simulink model "untitled"  (R2022b)
settings: Solver=ode15s  StartTime=0.0  StopTime=10  RelTol=1e-3
settings Model: Creator=Cmos  LastModifiedBy=Cmos

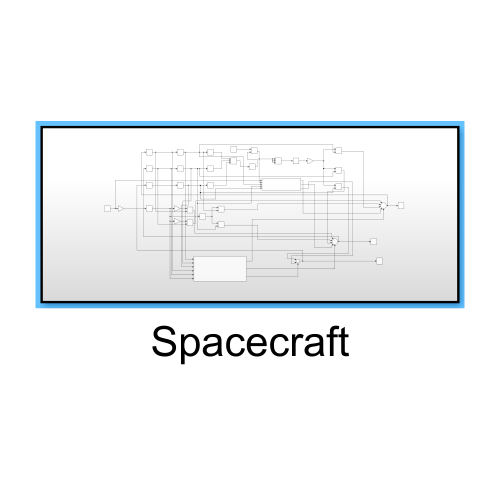
[thumbnail: Simulink's stored preview of the top-level diagram]
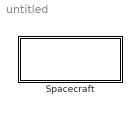
== system untitled ==
  Spacecraft : Subsystem

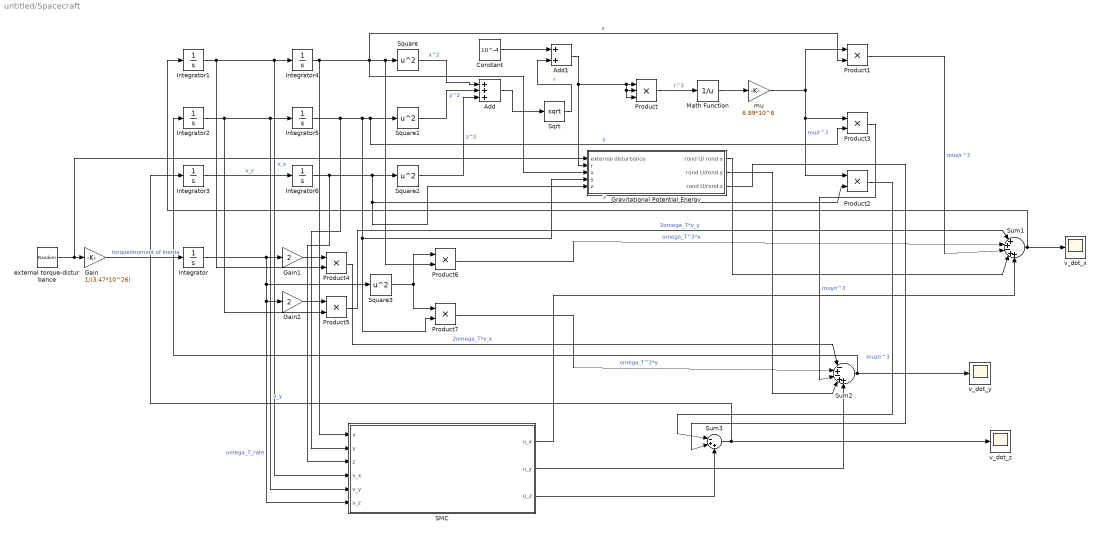
== system untitled/Spacecraft ==
  Add : Sum  Inputs=+++
  Add1 : Sum
  Constant : Constant  Value=10^-4
  Gain : Gain  Gain=1/(3.47*10^26)
  Gain1 : Gain  Gain=2
  Gain2 : Gain  Gain=2
  Gravitational Potential Energy : Subsystem
  Integrator : Integrator  InitialCondition=4.17*10^-6
  Integrator1 : Integrator
  Integrator2 : Integrator
  Integrator3 : Integrator
  Integrator4 : Integrator  InitialCondition=1
  Integrator5 : Integrator  InitialCondition=1
  Integrator6 : Integrator  InitialCondition=1
  Math Function : Math  Operator=reciprocal
  Product : Product  Inputs=3
  Product{1..7} (7 alike) : Product
  SMC : Subsystem
  Sqrt : Sqrt
  Square{,1..3} (4 alike) : Math  Operator=square
  Sum1 : Sum  Inputs=|++-++
  Sum2 : Sum  Inputs=|-+-++
  Sum3 : Sum  Inputs=|-++
  external torque-disturbance : RandomNumber  Variance=10^-12  SampleTime=0.1
  mu : Gain  Gain=6.89*10^6
  v_dot_x : Scope
  v_dot_y : Scope
  v_dot_z : Scope
  wires:
  Integrator1/1 -> Integrator4/1, SMC/4(v_x), Product4/2  "v_x"
  Integrator2/1 -> Integrator5/1, SMC/5(v_y), Product5/2  "v_y"
  Integrator3/1 -> Integrator6/1  "v_z"
  Integrator4/1 -> Product6/2, Square/1, Product1/2, Gravitational Potential Energy/3(x), SMC/1(x)  "x"
  Integrator5/1 -> SMC/2(y), Product7/2, Gravitational Potential Energy/4(y), Square1/1, Product3/2  "y"
  Integrator6/1 -> Product2/2, Gravitational Potential Energy/5(z), Square2/1, SMC/3(z)  "z"
  Square/1 -> Add/1  "x^2"
  Square1/1 -> Add/2  "y^2"
  Square2/1 -> Add/3  "z^2"
  Product/1 -> Math Function/1  "r^3"
  Math Function/1 -> mu/1
  mu/1 -> Product1/1, Product2/1, Product3/1  "mu/r^3"
  Product1/1 -> Sum1/3  "mux/r^3"
  Product3/1 -> Sum2/3  "muy/r^3"
  Product2/1 -> Sum3/1  "muz/r^3"
  external torque-disturbance/1 -> Gravitational Potential Energy/1(external disturbance), Gain/1
  Gain/1 -> Integrator/1  "torque/moment of inertia"
  Integrator/1 -> SMC/6(v_z), Gain2/1, Square3/1, Gain1/1  "omega_T_rate"
  Square3/1 -> Product7/1, Product6/1
  Gain1/1 -> Product4/1
  Gain2/1 -> Product5/1
  Product5/1 -> Sum1/1  "2omega_T*v_y"
  Product6/1 -> Sum1/2  "omega_T^2*x"
  Product7/1 -> Sum2/2  "omega_T^2*y"
  Gravitational Potential Energy/1(rond U/ rond x) -> Sum1/4
  Sum1/1 -> Integrator1/1, v_dot_x/1
  Product4/1 -> Sum2/1  "2omega_T*v_x"
  Gravitational Potential Energy/2(rond U/rond y) -> Sum2/4
  Sum2/1 -> Integrator2/1, v_dot_y/1
  Gravitational Potential Energy/3(rond U/rond z) -> Sum3/2
  Sum3/1 -> Integrator3/1, v_dot_z/1
  Constant/1 -> Add1/1
  Add/1 -> Sqrt/1
  Sqrt/1 -> Add1/2  "r"
  Add1/1 -> Gravitational Potential Energy/2(r), Product/2, Product/3, Product/1
  SMC/3(u_z) -> Sum3/3
  SMC/2(u_y) -> Sum2/5
  SMC/1(u_x) -> Sum1/5

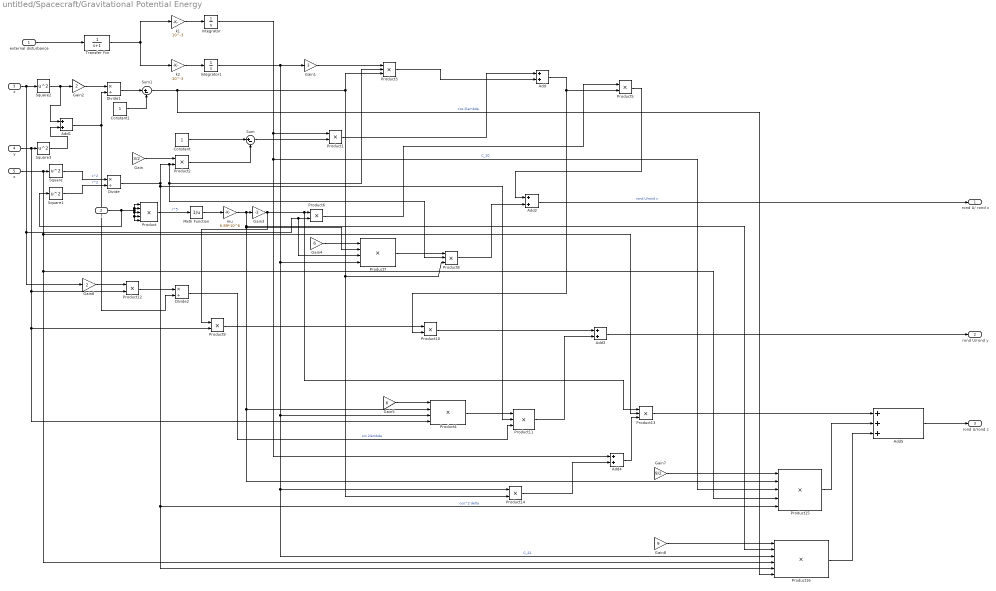
== system untitled/Spacecraft/Gravitational Potential Energy ==
  external disturbance : Inport
  r : Inport  Port=2
  x : Inport  Port=3
  y : Inport  Port=4
  z : Inport  Port=5
  Add{,1..4} (5 alike) : Sum
  Add5 : Sum  Inputs=+++
  Constant : Constant
  Constant1 : Constant
  Divide : Product  Inputs=*/
  Divide1 : Product  Inputs=*/
  Divide2 : Product  Inputs=*/
  Gain : Gain  Gain=3/2
  Gain1 : Gain  Gain=3
  Gain2 : Gain  Gain=2
  Gain3 : Gain  Gain=-3
  Gain4 : Gain  Gain=6
  Gain5 : Gain  Gain=6
  Gain6 : Gain  Gain=2
  Gain7 : Gain  Gain=9/2
  Gain8 : Gain  Gain=9
  Integrator : Integrator  InitialCondition=-0.1
  Integrator1 : Integrator  InitialCondition=0.02
  Math Function : Math  Operator=reciprocal
  Product : Product  Inputs=5
  Product{1..2,5..6,9..10,12,14} (8 alike) : Product
  Product{3,8,11,13} (4 alike) : Product  Inputs=3
  Product15 : Product  Inputs=5
  Product16 : Product  Inputs=6
  Product4 : Product  Inputs=4
  Product7 : Product  Inputs=4
  Square{,1..3} (4 alike) : Math  Operator=square
  Sum : Sum  Inputs=|+-
  Sum1 : Sum  Inputs=|+-
  Transfer Fcn : TransferFcn  Denominator=[1 1]
  k1 : Gain  Gain=10^-3
  k2 : Gain  Gain=10^-3
  mu : Gain  Gain=6.89*10^6
  rond U/ rond x : Outport
  rond U/rond y : Outport  Port=2
  rond U/rond z : Outport  Port=3
  wires:
  Integrator/1 -> Add4/1, Product15/3, Product1/1  "C_20"
  Integrator1/1 -> Product16/3, Product14/1, Product4/3, Product7/4, Gain1/1  "C_22"
  k1/1 -> Integrator/1
  k2/1 -> Integrator1/1
  r/1 -> Square1/1, Product/5, Product/4, Product/3, Product/1, Product/2
  Product/1 -> Math Function/1  "r^5"
  Math Function/1 -> mu/1
  mu/1 -> Product15/2, Product4/2, Product7/2, Product16/2, Gain3/1
  Gain3/1 -> Product9/1, Product13/1, Product6/1
  z/1 -> Product16/4, Product15/4, Product13/2, Square/1
  Square/1 -> Divide/1  "z^2"
  Square1/1 -> Divide/2  "r^2"
  Gain/1 -> Product2/1
  Divide/1 -> Product16/5, Product15/5, Product11/2, Product3/2, Product8/2, Product2/2  "cos^2 delta"
  Constant/1 -> Sum/1
  Product2/1 -> Sum/2
  x/1 -> Product6/2, Product7/3, Gain6/1, Square2/1
  y/1 -> Product9/2, Product4/4, Product12/2, Square3/1
  Square2/1 -> Add1/1, Gain2/1
  Gain2/1 -> Divide1/1
  Square3/1 -> Add1/2
  Add1/1 -> Divide2/2, Divide1/2
  Divide1/1 -> Sum1/1
  Constant1/1 -> Sum1/2
  Sum1/1 -> Product16/6, Product8/3, Product14/2, Product3/3  "cos 2lambda"
  Sum/1 -> Product1/2
  Gain1/1 -> Product3/1
  Product1/1 -> Add/1
  Product6/1 -> Product5/1
  Add/1 -> Product10/2, Product5/2
  Gain4/1 -> Product7/1
  Product7/1 -> Product8/1
  Product5/1 -> Add2/1
  Product8/1 -> Add2/2
  Add2/1 -> rond U/ rond x/1  "rond U/rond x"
  Product9/1 -> Product10/1
  Product3/1 -> Add/2
  Product10/1 -> Add3/1
  Gain5/1 -> Product4/1
  Product4/1 -> Product11/1
  Gain6/1 -> Product12/1
  Product12/1 -> Divide2/1
  Divide2/1 -> Product11/3  "sin 2lambda"
  Product11/1 -> Add3/2
  Add3/1 -> rond U/rond y/1
  Product14/1 -> Add4/2
  Add4/1 -> Product13/3
  Product13/1 -> Add5/1
  Add5/1 -> rond U/rond z/1
  Gain7/1 -> Product15/1
  Product15/1 -> Add5/2
  Gain8/1 -> Product16/1
  Product16/1 -> Add5/3
  external disturbance/1 -> Transfer Fcn/1
  Transfer Fcn/1 -> k2/1, k1/1

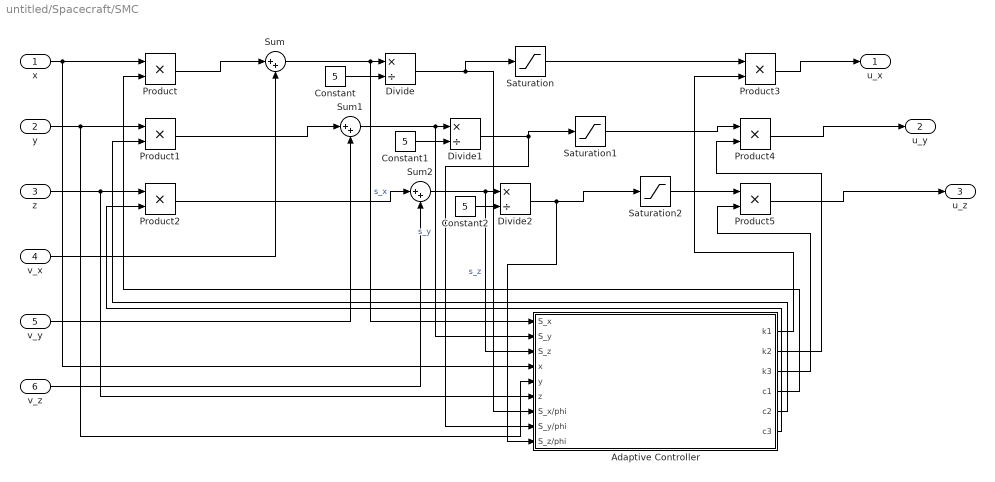
== system untitled/Spacecraft/SMC ==
  x : Inport
  y : Inport  Port=2
  z : Inport  Port=3
  v_x : Inport  Port=4
  v_y : Inport  Port=5
  v_z : Inport  Port=6
  Adaptive Controller : Subsystem
  Constant : Constant  Value=5
  Constant1 : Constant  Value=5
  Constant2 : Constant  Value=5
  Divide : Product  Inputs=*/
  Divide1 : Product  Inputs=*/
  Divide2 : Product  Inputs=*/
  Product{,1..5} (6 alike) : Product
  Saturation : Saturate  UpperLimit=+1  LowerLimit=-1
  Saturation1 : Saturate  UpperLimit=+1  LowerLimit=-1
  Saturation2 : Saturate  UpperLimit=+1  LowerLimit=-1
  Sum : Sum  Inputs=|++
  Sum1 : Sum  Inputs=|++
  Sum2 : Sum  Inputs=|++
  u_x : Outport
  u_y : Outport  Port=2
  u_z : Outport  Port=3
  wires:
  x/1 -> Product/1, Adaptive Controller/4(x)
  Product/1 -> Sum/1
  v_x/1 -> Sum/2
  y/1 -> Product1/1, Adaptive Controller/5(y)
  Product1/1 -> Sum1/1
  v_y/1 -> Sum1/2
  z/1 -> Product2/1, Adaptive Controller/6(z)
  Product2/1 -> Sum2/1
  v_z/1 -> Sum2/2
  Saturation2/1 -> Product5/1
  Saturation1/1 -> Product4/1
  Saturation/1 -> Product3/1
  Product3/1 -> u_x/1
  Product4/1 -> u_y/1
  Product5/1 -> u_z/1
  Sum/1 -> Adaptive Controller/1(S_x), Divide/1  "s_x"
  Sum2/1 -> Adaptive Controller/3(S_z), Divide2/1  "s_z"
  Sum1/1 -> Adaptive Controller/2(S_y), Divide1/1  "s_y"
  Constant/1 -> Divide/2
  Divide/1 -> Saturation/1, Adaptive Controller/7(S_x/phi)
  Constant1/1 -> Divide1/2
  Divide1/1 -> Saturation1/1, Adaptive Controller/8(S_y/phi)
  Constant2/1 -> Divide2/2
  Divide2/1 -> Saturation2/1, Adaptive Controller/9(S_z/phi)
  Adaptive Controller/4(c1) -> Product/2
  Adaptive Controller/5(c2) -> Product1/2
  Adaptive Controller/6(c3) -> Product2/2
  Adaptive Controller/1(k1) -> Product3/2
  Adaptive Controller/2(k2) -> Product4/2
  Adaptive Controller/3(k3) -> Product5/2

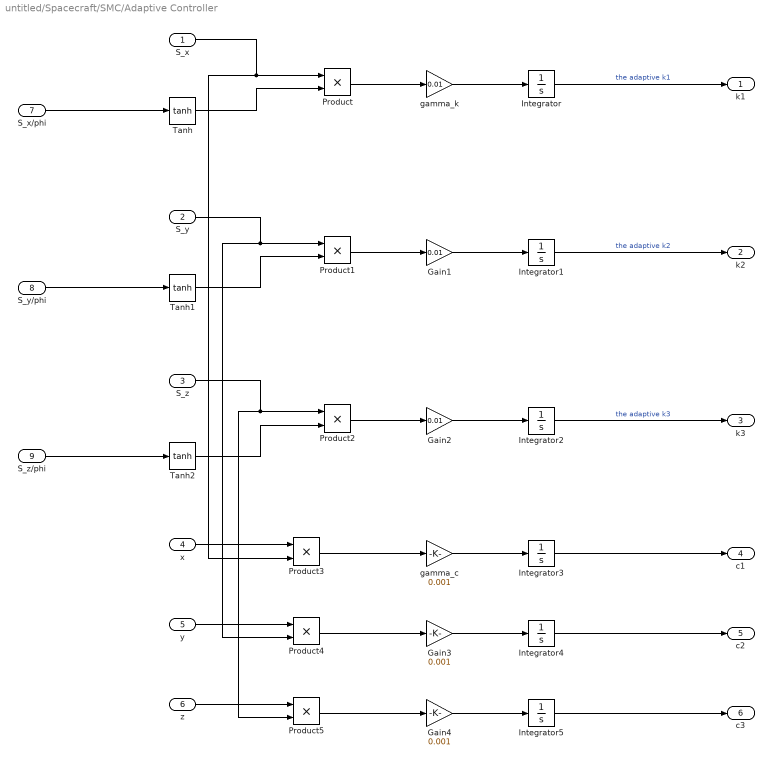
== system untitled/Spacecraft/SMC/Adaptive Controller ==
  S_x : Inport
  S_y : Inport  Port=2
  S_z : Inport  Port=3
  x : Inport  Port=4
  y : Inport  Port=5
  z : Inport  Port=6
  S_x/phi : Inport  Port=7
  S_y/phi : Inport  Port=8
  S_z/phi : Inport  Port=9
  Gain1 : Gain  Gain=0.01
  Gain2 : Gain  Gain=0.01
  Gain3 : Gain  Gain=0.001
  Gain4 : Gain  Gain=0.001
  Integrator : Integrator  InitialCondition=-10
  Integrator1 : Integrator  InitialCondition=-10
  Integrator2 : Integrator  InitialCondition=-10
  Integrator3 : Integrator  InitialCondition=4
  Integrator4 : Integrator  InitialCondition=4
  Integrator5 : Integrator  InitialCondition=4
  Product{,1..5} (6 alike) : Product
  Tanh : Trigonometry  Operator=tanh
  Tanh1 : Trigonometry  Operator=tanh
  Tanh2 : Trigonometry  Operator=tanh
  gamma_c : Gain  Gain=0.001
  gamma_k : Gain  Gain=0.01
  k1 : Outport
  k2 : Outport  Port=2
  k3 : Outport  Port=3
  c1 : Outport  Port=4
  c2 : Outport  Port=5
  c3 : Outport  Port=6
  wires:
  S_x/1 -> Product/1, Product3/2
  Tanh/1 -> Product/2
  S_y/1 -> Product1/1, Product4/2
  Tanh1/1 -> Product1/2
  S_z/1 -> Product2/1, Product5/2
  Tanh2/1 -> Product2/2
  Product/1 -> gamma_k/1
  Product1/1 -> Gain1/1
  Product2/1 -> Gain2/1
  gamma_k/1 -> Integrator/1
  Gain1/1 -> Integrator1/1
  Gain2/1 -> Integrator2/1
  Integrator/1 -> k1/1  "the adaptive k1"
  Integrator1/1 -> k2/1  "the adaptive k2"
  Integrator2/1 -> k3/1  "the adaptive k3"
  x/1 -> Product3/1
  y/1 -> Product4/1
  z/1 -> Product5/1
  Product3/1 -> gamma_c/1
  Product4/1 -> Gain3/1
  Product5/1 -> Gain4/1
  gamma_c/1 -> Integrator3/1
  Gain3/1 -> Integrator4/1
  Gain4/1 -> Integrator5/1
  Integrator3/1 -> c1/1
  Integrator4/1 -> c2/1
  Integrator5/1 -> c3/1
  S_x/phi/1 -> Tanh/1
  S_y/phi/1 -> Tanh1/1
  S_z/phi/1 -> Tanh2/1
